simulink model "mconversion14"  (Simulink 6.0)
settings: Solver=ode3  StartTime=0.0  StopTime=10.0  RelTol=1e-3
settings Model: Creator=awarlock  LastModifiedBy=awarlock  ExtModeAutoUpdateStatusClock=off
settings OptimizationCC: InlineParams=on
settings DebuggingCC: CheckExecutionContextPreStartOutputMsg=on  CheckExecutionContextRuntimeOutputMsg=on
settings SFSimCC: SFSimApplyToAllLibs=on  SFSimBuildMode=Incremental

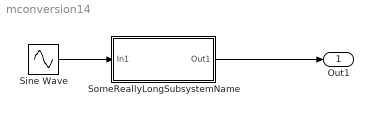
== system mconversion14 ==
  Sine Wave : Sin  SampleTime=0
  SomeReallyLongSubsystemName : Subsystem  TreatAsAtomicUnit=on  PropExecContextAcrossSSBoundary=on
  Out1 : Outport
  wires:
  Sine Wave/1 -> SomeReallyLongSubsystemName/1(In1)
  SomeReallyLongSubsystemName/1(Out1) -> Out1/1

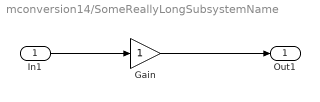
== system mconversion14/SomeReallyLongSubsystemName ==
  In1 : Inport  LatchInput=off
  Gain : Gain
  Out1 : Outport
  wires:
  In1/1 -> Gain/1
  Gain/1 -> Out1/1
